simulink model "Electrical787_Isolated_2013a"  (R2013a)
settings: Solver=ode45  StartTime=0.0  StopTime=1000  RelTol=1e-3
libraries: PowerFlowLib x27, simulink x4
(part 1 of 2)
settings Model: CovModelRefEnable=off  Creator=Andrew  LastModifiedBy=Andrew
settings DataIOCC: SaveFormat=StructureWithTime
settings DebuggingCC: UnderspecifiedInitializationDetection=Simplified  MergeDetectMultiDrivingBlocksExec=error  SolverPrmCheckMsg=none  FrameProcessingCompatibilityMsg=error  StateNameClashWarn=none
settings HardwareCC: ProdBitPerPointer=64  ProdLargestAtomicFloat=Float  ProdIntDivRoundTo=Zero  ProdEndianess=LittleEndian  ProdHWDeviceType=Specified
settings GRTTargetCC: CodeReplacementLibrary=C89/C90 (ANSI)  GeneratePreprocessorConditionals=Use local settings

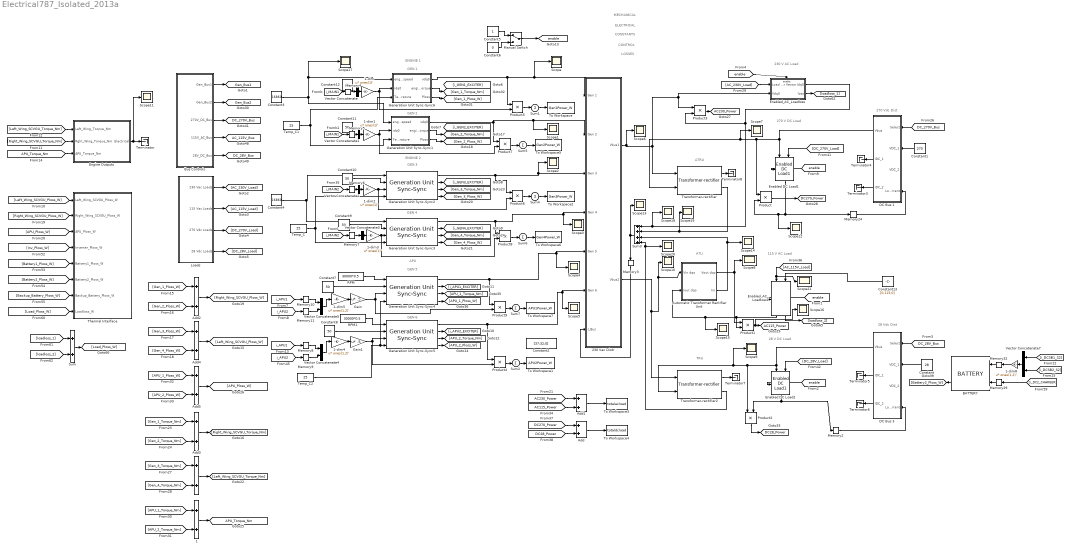
== system Electrical787_Isolated_2013a ==
  note: GEN 1
  note: ENGINE 1
  note: GEN 2
  note: GEN 3
  note: ENGINE 2
  note: GEN 4
  note: GEN 5
  note: APU
  note: GEN 6
  note: ATRU
  note: TRU
  note: 230 V AC Load
  note: 270 Vdc Dist
  note: 28 Vdc Dist
  note: 270 V DC Load
  note: CONSTANTS
  note: CONTROL
  note: LOSSES
  note: MECHANICAL
  note: ELECTRICAL
  note: ATU
  note: 115 V AC Load
  note: 28 V DC Load
  " " : Sum
  " 1" : Sum
  1-dim{,1..3} (4 alike) : Gain  Gain=ones(1)'  Multiplication=Matrix(u*K)
  1-dim4 : Gain  Gain=ones(1,2)'  Multiplication=Matrix(u*K)
  1-dim5 : Gain  Gain=ones(1,2)'  Multiplication=Matrix(u*K)
  1-dim8 : Gain  Gain=ones(1,2)'  Multiplication=Matrix(u*K)
  230 Vac Distr : Subsystem
  Add{,1..5} (6 alike) : Sum
  Automatic Transformer Rectifier Unit : Subsystem
  BATTERY : PowerFlowLib/Energy & Power Systems/Electrical/Battery/BATTERY  NO_CELLS=9  NO_MODULES=10  INITIAL_SOC=1
  Bus Controls : Subsystem  mask{BUS1=Generator 1, BUS2=Generator 2, MBUS1=Generator Bus 1, ACTBUS1=Generator Bus 1, MBUS2=Generator Bus 2, ACTBUS2=Generator Bus 2, IDCBUS1=Battery 1, IDCBUS2=Battery 2}
      mask prompts: BUS1 "Source for Bus 1"; BUS2 "Source for Bus 2"; MBUS1 "Load on Main Bus 1 drawn from"; ACTBUS1 "Load on AC Transfer Bus 1 drawn from"; MBUS2 "Load on Main Bus 2 drawn from"; ACTBUS2 "Load on AC Transfer Bus 2 drawn from"; IDCBUS1 "Source for DC Service Bus 1"; IDCBUS2 "Source for DC Service Bus 2"
      mask help:
      | Specify the source from which different buses receive power. There are
      | 1. Two Generator buses (Bus 1-2)
      | 2. Two AC Main buses (Main Bus 1-2))
      | 3. Two AC Transfer buses and (AC Transfer Bus 1-2)
      | 4. Two DC Intermediate buses (DC Intermediate Bus 1-2)
      mask init:
      | switch BUS1
      |     case 1
      |         BUS1CONTROL = 1;
      |     case 2
      |         BUS1CONTROL = 2;
      |     case 3
      |         BUS1CONTROL = 3;
      |     case 4
      |         BUS1CONTROL = 4;
      | end
      | 
      | switch BUS2
      |     case 1
      |         BUS2CONTROL = 1;
      |     case 2
      |         BUS2CONTROL = 2;
      |     case 3
      |         BUS2CONTROL = 3;
      |     case 4
      |         BUS2CONTROL = 4;
      | end
      | 
      | switch MBUS1
      |     case 1
      |         MBUS1CONTROL = 1;
      |     case 2
      |         MBUS1CONTROL = 2;
      | end
      | 
      | switch ACTBUS1
      |     case 1
      |         ACTBUS1CONTROL = 1;
      |     case 2
      |         ACTBUS1CONTROL = 2;
      | end
      | 
      | switch MBUS2
      |     case 1
      |         MBUS2CONTROL = 1;
      |     case 2
      |         MBUS2CONTROL = 2;
      | end
      | 
      | switch ACTBUS2
      |     case 1
      |         ACTBUS2CONTROL = 1;
      |     case 2
      |         ACTBUS2CONTROL = 2;
      | end
      | 
      | switch IDCBUS1
      |     case 1
      |         IDCBUS1CONTROL = 1;
      |     case 2
      |         IDCBUS1CONTROL = 2;
      | end
      | 
      | switch IDCBUS2
      |     case 1
      |         IDCBUS2CONTROL = 1;
      |     case 2
      |         IDCBUS2CONTROL = 2;
      | end
      mask TypeOptions BUS1: Generator 1  | APU  | GND | AUX SUPPLY
      mask TypeOptions BUS2: Generator 2  | APU  | GND | AUX SUPPLY
      mask TypeOptions MBUS1: Generator Bus 1 | Generator Bus 2
      mask TypeOptions ACTBUS1: Generator Bus 1 | Generator Bus 2
      mask TypeOptions MBUS2: Generator Bus 1 | Generator Bus 2
      mask TypeOptions ACTBUS2: Generator Bus 1 | Generator Bus 2
      mask TypeOptions IDCBUS1: Battery 1 | Battery 2
      mask TypeOptions IDCBUS2: Battery 1 | Battery 2
  Constant : Constant  Value=28
  Constant1 : Constant  Value=270
  Constant{7..12} (6 alike) : Constant  Value=50
  Constant13 : Constant  Value=[0,115,0]
  Constant2 : Constant  Value=[37;32;0]
  Constant3 : Constant  Value=16860
  Constant4 : Constant  Value=16860
  Constant5 : Constant
  Constant6 : Constant  Value=0
  DC Bus 1 : Subsystem  mask(DC Service Bus){}
      mask help: Service Bus
  DC Bus 3 : Subsystem  mask(DC Service Bus){}
      mask help: Service Bus
  Enabled DC Load1 : PowerFlowLib/Energy & Power Systems/Electrical/Loads/Enabled  DC Load1
  Enabled DC Load2 : PowerFlowLib/Energy & Power Systems/Electrical/Loads/Enabled  DC Load1
  Enabled_AC_Loadloss : Subsystem  AncestorBlock=PowerFlowLib/Energy & Power Systems/Electrical/Loads/Enabled_AC_Loadloss  mask(AC Loads){P=500, PF=0.85, ILRMS=0, R=10000, X=10000}
      mask prompts: P "Real Power (W)"; PF "Power factor (Range: 0 -1) : Prefix '-' sign for Cap loads"; ILRMS "Current Loading"; R "Resistance (Ohms)"; X "Reactance (Ohms)"
      mask help:
      | Enabled AC Load System.
      | Note:
      | Load Master Vector input is 1x3 matrix representing (P[W] Q[Var] I[A])
      | Extra load can be input in the boxes below and will be added with the Load Master Vector.
      mask Help: eval('open(''AC Loads_help.html'')');
      mask Callback PF:
      | blk = gcb;
      | PF    = str2num(get_param(blk,'PF'));
      | 
      | if ((PF>1) | (PF<-1))
      |    g = warndlg('Power factor magnitude should be between 0 and 1 . Reverting to default value 1','Error1','CreateMode');
      |    set_param(blk,'PF','1');
      |    open_system(blk,'mask');
      | end
      | 
      | clear g PF blk
      mask Callback X:
      | blk = gcb;
      | value1 = str2num(get_param(blk,'R'));
      | value2 = str2num(get_param(blk,'X'));
      | % eff    = str2num(get_param(blk,'E'));
      | 
      | if (value1==0) && (value2==0)
      |   h = warndlg('Both R and X cannot be 0. Reverting to default values','Error','CreateMode');
      |   set_param(blk,'R','10000');
      |   set_param(blk,'X','10000');
      | %   if ishandle(h)
      | %       close(h)
      |   open_system(blk,'mask');
      | end
      | 
      | % if ((eff>1) | (eff<0))
      | %    g = warndlg('Efficiency should be between 0 and 1 . Reverting to default value 1','Error1','CreateMode');
      | %    set_param(blk,'E','1');
      | %    open_system(blk,'mask');
      | % end
      | 
      | clear h eff blk value1 value2
      mask Display:
      | %image(imread('ACload.png'))
      | 
      | % port_label('input',1,'{\bf EXT LOAD VECTOR}','TexMode','on')
      | % port_label('input',2,'{\bf Vdq0}','TexMode','on')
      | %
      | % port_label('output',1,'{\bf Idq0}','TexMode','on')
      | % port_label('output',2,'{\bf PLOSS}','TexMode','on')
      | 
      | image(imread('ACloads.png'))
      | 
      | port_label('input',1,'{\bf Load}','TexMode','on')
      | port_label('input',2,'{\bf V_d_q_0}','TexMode','on')
      | port_label('Enable','{\bf switch}','Texmode','on')
      | 
      | port_label('output',1,'{\bf I_d_q_0}','TexMode','on')
      | port_label('output',2,'{\bf P_l_o_s_s}','TexMode','on')
  Enabled_AC_Loadloss1 : PowerFlowLib/Energy & Power Systems/Electrical/Loads/Enabled_AC_Loadloss  P=500  PF=0.85  ILRMS=0  R=10000  X=10000
  Engine Outputs : Subsystem
  Gain : Gain  Gain=.5  Multiplication=Matrix(u*K)
  Gain1 : Gain  Gain=.5  Multiplication=Matrix(u*K)
  Generation Unit Sync-Sync1 : Subsystem  AncestorBlock=PowerFlowLib/Energy & Power Systems/Electrical/Systems/Generation Unit Sync-Sync  mask{machine_mode=100kVA_Gen, Rs=0.0163, Xls=0.00054, Xmd=0.66176, Xmq=0.00099, R_fd=0.016, Xlfd=0.2092, R_1d=0.2047, Xl1d=0.6524, R_1q=0.0429, R_2q=0.0429, Xl1q=0.0639, Xl2q=0.0639, ws=377, RTL=0.001, XTL=0.1, KA=20, KF=0.063, T_f=0.35, TA=0.2, KE=1, TE=0.314, SB=100000, VBDQ=100, wB=377, P=6, H=0.1777, R_conv_gen=0.05, mc_gen=10000, Vnom=115, fan_load='init_fan_characteristics.mat', exciter_param='exciter.mat'}
      mask prompts: machine_mode "Machine Preset"; Rs "Stator Resistance [ohm]"; Xls "Stator Leakage Reactance [ohm]"; Xmd "Magnetizing Direct Axis Reactance [ohm]"; Xmq "Magnetizing Quadrature Axis Reactance [ohm]"; R_fd "Field Resistance [ohm]"; Xlfd "Field Leakage Reactance [ohm]"; R_1d "Transient Direct Axis Resistance [ohm]"; Xl1d "Transient Leakage Direct Axis Reactance [ohm]"; R_1q "Transient Quadrature Axis Resistance [ohm]"; R_2q "Subtransient Quadrature Axis Resistance [ohm]"; Xl1q "Transient Leakage Quadrature Axis Reactance [ohm]"; Xl2q "Subtransient Leakage Quadrature Axis Reactance [ohm]"; ws "Rotational Speed [rad/s]"; RTL "Resistance [ohm]"; XTL "Reactance [ohm]"; SB "Baes Complex Power [VA]"; VBDQ "Base Direct and Quadrature Axis Armature Voltage [V]"; wB "Base Electrical Frequency [rad/s]"; P "Number of Pole Pairs"; H "Shaft Inertia Constant [s]"; Vnom "Nominal Voltage [V]"; fan_load "Fan Load"; exciter_param "Exciter Machine Parameters"
      mask help:
      | A generator system block implements a generic power generation unit consisting of a gearbox, a synchronous generator, a synchronous exciter and exciter controls.
      | The generator size can be selected from the drop window below.
      | (For advanced-users) When the User-defined option is selected from the drop window, the generator parameters can be manually specified in the tabs below.
      |
      | Block Inputs:
      |
      | #1: Jet engine low pressure spool [RPM]
      | #2: Exciter system supply voltage [V]
      | #3: Synchronous reference frame line currents  [A]
      |
      | Block Output:
      |
      | #1: Synchronous reference frame line voltages [V]
      | #2: Exciter system supply current [A]
      | #3: Electromagnetic torque on the low pressure spool  [N-M]
      | #4: Heat rejected to the cooling system or ambient [W]
      mask init:
      | load(fan_load);
      | 
      | % Inductances
      | Xd = Xls + Xmd;
      | Xq = Xls + Xmq;
      | Xfd = Xlfd + Xmd;
      | X1q = Xl1q + Xmq;
      | Xd1 = Xd - Xmd^2/Xfd;
      | Xq1 = Xq - Xmq^2/X1q;
      | Xd2 = Xls + (1/(1/Xmd + 1/Xlfd + 1/Xl1d));
      | Xq2 = Xls + (1/(1/Xmq + 1/Xl1q + 1/Xl2q));
      | Tdo1 = Xfd/ws/R_fd;
      | Tqo1 = X1q/ws/R_1q;
      | Tdo2 = 1/ws/R_1d*(Xl1d + 1/(1/Xmd + 1/Xlfd));
      | Tqo2 = 1/ws/R_2q*(Xl2q+1/(1/Xmq + 1/Xl1q));
      | 
      | % Base Quantities
      | 
      | TB = (P/2)*SB/wB;
      | IBDQ = SB/VBDQ;
      | LBDQ = VBDQ/wB;
      | 
      | IBFD = IBDQ;
      | IB1D = IBDQ;
      | IB1Q = IBDQ;
      | IB2Q = IBDQ;
      | 
      | VBFD = SB/IBFD;
      | VB1D = SB/IB1D;
      | VB1Q = SB/IB1Q;
      | VB2Q = SB/IB2Q;
      | 
      | LBFD = VBFD/wB;
      | LB1D = VB1D/wB;
      | LB1Q = VB1Q/wB;
      | LB2Q = VB2Q/wB;
      | 
      | J = 2*H/(wB*2/P)^2*SB;
      | M = 2*H/wB;
      | 
      | % Exciter
      | 
      | data_exc = load(exciter_param);
      |   
      | % Stator
      | Rs_exc = data_exc.r(1);
      | Xls_exc = data_exc.r(2);
      | Xmd_exc = data_exc.r(3);
      | Xmq_exc = data_exc.r(4);
      | 
      | % Field
      | R_fd_exc = data_exc.r(5);
      | Xlfd_exc = data_exc.r(6);
      | % Dampers
      | R_1d_exc = data_exc.r(7);
      | Xl1d_exc = data_exc.r(8);
      | R_1q_exc = data_exc.r(9);
      | Xl1q_exc = data_exc.r(10);
      | R_2q_exc = data_exc.r(11);
      | Xl2q_exc = data_exc.r(12);
      | 
      | % Rotor
      | P_exc = data_exc.r(13);
      | ws_exc = data_exc.r(14);
      | 
      | % Inductances
      | Xd_exc = Xls_exc + Xmd_exc;
      | Xq_exc = Xls_exc + Xmq_exc;
      | Xfd_exc = Xlfd_exc + Xmd_exc;
      | X1q_exc = Xl1q_exc + Xmq_exc;
      | Xd1_exc = Xd_exc - Xmd_exc^2/Xfd_exc;
      | Xq1_exc = Xq_exc - Xmq_exc^2/X1q_exc;
      | Xd2_exc = Xls_exc + (1/(1/Xmd_exc + 1/Xlfd_exc + 1/Xl1d_exc));
      | Xq2_exc = Xls_exc + (1/(1/Xmq_exc + 1/Xl1q_exc + 1/Xl2q_exc));
      | Tdo1_exc = Xfd_exc/ws_exc/R_fd_exc;
      | Tqo1_exc = X1q_exc/ws_exc/R_1q_exc;
      | Tdo2_exc = 1/ws_exc/R_1d_exc*(Xl1d_exc + 1/(1/Xmd_exc + 1/Xlfd_exc));
      | Tqo2_exc = 1/ws_exc/R_2q_exc*(Xl2q_exc+1/(1/Xmq_exc + 1/Xl1q_exc));
      | 
      | % Transmission Line
      | RTL_exc = data_exc.r(15);
      | XTL_exc = data_exc.r(16);
      | 
      | % Regulator and Governor
      | KA_exc = data_exc.r(17);
      | KF_exc = data_exc.r(18);
      | T_f_exc = data_exc.r(19);
      | TA_exc = data_exc.r(20);
      | KE_exc = data_exc.r(21);
      | TE_exc = data_exc.r(22);
      | 
      | % Base Quantities
      | SB_exc = data_exc.r(23);
      | VBDQ_exc = data_exc.r(24);
      | wB_exc = data_exc.r(25);
      | P_exc = data_exc.r(13);
      | H_exc = data_exc.r(26);
      | 
      | TB_exc = (P/2)*SB_exc/wB_exc;
      | IBDQ_exc = SB_exc/VBDQ_exc;
      | LBDQ_exc = VBDQ_exc/wB_exc;
      | 
      | IBFD_exc = IBDQ_exc;
      | IB1D_exc = IBDQ_exc;
      | IB1Q_exc = IBDQ_exc;
      | IB2Q_exc = IBDQ_exc;
      | 
      | VBFD_exc = SB_exc/IBFD_exc;
      | VB1D_exc = SB_exc/IB1D_exc;
      | VB1Q_exc = SB_exc/IB1Q_exc;
      | VB2Q_exc = SB_exc/IB2Q_exc;
      | 
      | LBFD_exc = VBFD_exc/wB_exc;
      | LB1D_exc = VB1D_exc/wB_exc;
      | LB1Q_exc = VB1Q_exc/wB_exc;
      | LB2Q_exc = VB2Q_exc/wB_exc;
      | 
      | J_exc = 2*data_exc.r(26)/(wB_exc*2/P_exc)^2*SB_exc;
      | M_exc = 2*H_exc/wB_exc;
      | 
      | R_conv_gen_exc = 1/data_exc.r(27);
      | mc_gen_exc = data_exc.r(28);
      mask Help: eval('open(''Generator System_help.html'')');
      mask TypeOptions machine_mode: 20kVA_Gen | 52.5kVA_Gen | 100kVA_Gen | 300kVA_Gen | 800kVA_Gen | 1MVA_Gen | User-defined
      mask Callback machine_mode:
      | h=get_param(gcb,'handle');
      | hblock=get(h);
      | data=load('GenProp.mat');
      | 
      | if strcmp(hblock.machine_mode,'User-defined')==1;
      |     adv_warn=warndlg(sprintf('User-defined parameters may lead to an unstable build.'));
      | 
      |     % grabs current values of enabled GUI parameters
      |     mskenabl = get_param(gcb,'MaskEnables');
      |     mskenabl(1:size(mskenabl,1)) = {'on'};  % sets all parameters to enable
      |     set_param(gcb,'MaskEnables',mskenabl)
      | 
      | else
      |     % For each generator preset references a column from GenProp.mat
      |     if strcmp(hblock.machine_mode,'20kVA_Gen')==1; n=1;
      |     elseif strcmp(hblock.machine_mode,'52.5kVA_Gen')==1; n=2;
      |     elseif strcmp(hblock.machine_mode,'100kVA_Gen')==1; n=3;
      |     elseif strcmp(hblock.machine_mode,'300kVA_Gen')==1; n=4;
      |     elseif strcmp(hblock.machine_mode,'800kVA_Gen')==1; n=5;
      |     elseif strcmp(hblock.machine_mode,'1MVA_Gen')==1; n=6;
      |     end
      |     % Set each parameter of the generator
      |     set1=num2str(data.r(1,n));
      |     set2=num2str(data.r(2,n));
      |     set3=num2str(data.r(3,n));
      |     set4=num2str(data.r(4,n));
      |     set_param(gcb,'Rs',set1,'Xls',set2,'Xmd',set3,'Xmq',set4)
      |     set1=num2str(data.r(5,n));
      |     set2=num2str(data.r(6,n));
      |     set_param(gcb,'R_fd',set1,'Xlfd',set2) %5 and 6
      |     set1=num2str(data.r(7,n));
      |     set2=num2str(data.r(8,n));
      |     set3=num2str(data.r(9,n));
      |     set4=num2str(data.r(10,n));
      |     set5=num2str(data.r(11,n));
      |     set6=num2str(data.r(12,n));
      |     set_param(gcb,'R_1d',set1,'Xl1d',set2,'R_1q',set3,'Xl1q',set4,'R_2q',set5,'Xl2q',set6) %7-12
      |     set1=num2str(data.r(14,n));
      |     set2=num2str(data.r(15,n));
      |     set3=num2str(data.r(16,n));
      |     set_param(gcb,'ws',set1,'RTL',set2,'XTL',set3)
      |     set1=num2str(data.r(17,n));
      |     set2=num2str(data.r(18,n));
      |     set3=num2str(data.r(19,n));
      |     set4=num2str(data.r(20,n));
      |     set5=num2str(data.r(21,n));
      |     set6=num2str(data.r(22,n));
      |     set_param(gcb,'KA',set1,'KF',set2,'T_f',set3,'TA',set4,'KE',set5,'TE',set6)
      |     set1=num2str(data.r(23,n));
      |     set2=num2str(data.r(24,n));
      |     set3=num2str(data.r(25,n));
      |     set4=num2str(data.r(13,n));
      |     set5=num2str(data.r(26,n));
      |     set_param(gcb,'SB',set1,'VBDQ',set2,'wB',set3,'P',set4,'H',set5)
      |     set1=num2str(1/data.r(27,n));
      |     set2=num2str(data.r(28,n));
      |     set_param(gcb,'R_conv_gen',set1,'mc_gen',set2)
      | 
      |     % grabs current values of enabled GUI parameters
      |     mskenabl = get_param(gcb,'MaskEnables');
      |     % sets all parameters to enable
      |     mskenabl(2:size(mskenabl,1)-3) = {'off'};
      |     set_param(gcb,'MaskEnables',mskenabl)
      | 
      | 
      | end
      | 
      | 
      | clear h hblock n data mskenabl
      | clear set1 set2 set3 set4 set5 set6
      mask Display:
      | image(imread('Generator.png')) % Load image
      | 
      | % Define inputs
      | 
      | port_label('input',1,'{\bf \omega_s_h_a_f_t}','Texmode','on')
      | port_label('input',2,'{\bf V_D_C}','Texmode','on')
      | port_label('input',3,'{\bf I_d_q_0}','Texmode','on')
      | port_label('input',4,'{\bf Temp}','Texmode','on')
      | 
      | % Define outputs
      | 
      | port_label('output',1,'{\bf V_d_q_0}','Texmode','on')
      | port_label('output',2,'{\bf I_D_C}','Texmode','on')
      | port_label('output',3,'{\bf \tau}','Texmode','on')
      | port_label('output',4,'{\bf P_l_o_s_s}','Texmode','on')
      | 
      | % % Define inputs
      | %
      | % port_label('input',1,'{\bf Generator Speed}','Texmode','on')
      | % port_label('input',2,'{\bf Battery Voltage}','Texmode','on')
      | % port_label('input',3,'{\bf Line Currents}','Texmode','on')
      | %
      | % % Define outputs
      | %
      | % port_label('output',1,'{\bf Line Voltages}','Texmode','on')
      | % port_label('output',2,'{\bf Battery Current}','Texmode','on')
      | % port_label('output',3,'{\bf Generator Torque}','Texmode','on')
      | % port_label('output',4,'{\bf Power Loss}','Texmode','on')
  Generation Unit Sync-Sync{2..5} (4 alike) : PowerFlowLib/Energy & Power Systems/Electrical/Systems/Generation Unit Sync-Sync  machine_mode=100kVA_Gen  Rs=0.0163  Xls=0.00054  Xmd=0.66176  Xmq=0.00099  R_fd=0.016  Xlfd=0.2092  R_1d=0.2047  Xl1d=0.6524  R_1q=0.0429  R_2q=0.0429  Xl1q=0.0639  Xl2q=0.0639  ws=377  RTL=0.001  XTL=0.1  KA=20  KF=0.063  T_f=0.35  TA=0.2  KE=1  TE=0.314  SB=100000  VBDQ=100  wB=377  P=6  H=0.1777  R_conv_gen=0.05  mc_gen=10000  Vnom=115  fan_load='init_fan_characteristics.mat'  exciter_param='exciter.mat'
  Generation Unit Sync-Sync6 : Subsystem  AncestorBlock=PowerFlowLib/Energy & Power Systems/Electrical/Systems/Generation Unit Sync-Sync  mask{machine_mode=100kVA_Gen, Rs=0.0163, Xls=0.00054, Xmd=0.66176, Xmq=0.00099, R_fd=0.016, Xlfd=0.2092, R_1d=0.2047, Xl1d=0.6524, R_1q=0.0429, R_2q=0.0429, Xl1q=0.0639, Xl2q=0.0639, ws=377, RTL=0.001, XTL=0.1, KA=20, KF=0.063, T_f=0.35, TA=0.2, KE=1, TE=0.314, SB=100000, VBDQ=100, wB=377, P=6, H=0.1777, R_conv_gen=0.05, mc_gen=10000, Vnom=115, fan_load='init_fan_characteristics.mat', exciter_param='exciter.mat'}
      mask prompts: machine_mode "Machine Preset"; Rs "Stator Resistance [ohm]"; Xls "Stator Leakage Reactance [ohm]"; Xmd "Magnetizing Direct Axis Reactance [ohm]"; Xmq "Magnetizing Quadrature Axis Reactance [ohm]"; R_fd "Field Resistance [ohm]"; Xlfd "Field Leakage Reactance [ohm]"; R_1d "Transient Direct Axis Resistance [ohm]"; Xl1d "Transient Leakage Direct Axis Reactance [ohm]"; R_1q "Transient Quadrature Axis Resistance [ohm]"; R_2q "Subtransient Quadrature Axis Resistance [ohm]"; Xl1q "Transient Leakage Quadrature Axis Reactance [ohm]"; Xl2q "Subtransient Leakage Quadrature Axis Reactance [ohm]"; ws "Rotational Speed [rad/s]"; RTL "Resistance [ohm]"; XTL "Reactance [ohm]"; SB "Baes Complex Power [VA]"; VBDQ "Base Direct and Quadrature Axis Armature Voltage [V]"; wB "Base Electrical Frequency [rad/s]"; P "Number of Pole Pairs"; H "Shaft Inertia Constant [s]"; Vnom "Nominal Voltage [V]"; fan_load "Fan Load"; exciter_param "Exciter Machine Parameters"
      mask help:
      | A generator system block implements a generic power generation unit consisting of a gearbox, a synchronous generator, a synchronous exciter and exciter controls.
      | The generator size can be selected from the drop window below.
      | (For advanced-users) When the User-defined option is selected from the drop window, the generator parameters can be manually specified in the tabs below.
      |
      | Block Inputs:
      |
      | #1: Jet engine low pressure spool [RPM]
      | #2: Exciter system supply voltage [V]
      | #3: Synchronous reference frame line currents  [A]
      |
      | Block Output:
      |
      | #1: Synchronous reference frame line voltages [V]
      | #2: Exciter system supply current [A]
      | #3: Electromagnetic torque on the low pressure spool  [N-M]
      | #4: Heat rejected to the cooling system or ambient [W]
      mask init: same as Electrical787_Isolated_2013a/Generation Unit Sync-Sync1
      mask Help: eval('open(''Generator System_help.html'')');
      mask TypeOptions machine_mode: 20kVA_Gen | 52.5kVA_Gen | 100kVA_Gen | 300kVA_Gen | 800kVA_Gen | 1MVA_Gen | User-defined
      mask Callback machine_mode:
      | h=get_param(gcb,'handle');
      | hblock=get(h);
      | data=load('GenProp.mat');
      | 
      | if strcmp(hblock.machine_mode,'User-defined')==1;
      |     adv_warn=warndlg(sprintf('User-defined parameters may lead to an unstable build.'));
      | 
      |     % grabs current values of enabled GUI parameters
      |     mskenabl = get_param(gcb,'MaskEnables');
      |     mskenabl(1:size(mskenabl,1)) = {'on'};  % sets all parameters to enable
      |     set_param(gcb,'MaskEnables',mskenabl)
      | 
      | else
      |     % For each generator preset references a column from GenProp.mat
      |     if strcmp(hblock.machine_mode,'20kVA_Gen')==1; n=1;
      |     elseif strcmp(hblock.machine_mode,'52.5kVA_Gen')==1; n=2;
      |     elseif strcmp(hblock.machine_mode,'100kVA_Gen')==1; n=3;
      |     elseif strcmp(hblock.machine_mode,'300kVA_Gen')==1; n=4;
      |     elseif strcmp(hblock.machine_mode,'800kVA_Gen')==1; n=5;
      |     elseif strcmp(hblock.machine_mode,'1MVA_Gen')==1; n=6;
      |     end
      |     % Set each parameter of the generator
      |     set1=num2str(data.r(1,n));
      |     set2=num2str(data.r(2,n));
      |     set3=num2str(data.r(3,n));
      |     set4=num2str(data.r(4,n));
      |     set_param(gcb,'Rs',set1,'Xls',set2,'Xmd',set3,'Xmq',set4)
      |     set1=num2str(data.r(5,n));
      |     set2=num2str(data.r(6,n));
      |     set_param(gcb,'R_fd',set1,'Xlfd',set2) %5 and 6
      |     set1=num2str(data.r(7,n));
      |     set2=num2str(data.r(8,n));
      |     set3=num2str(data.r(9,n));
      |     set4=num2str(data.r(10,n));
      |     set5=num2str(data.r(11,n));
      |     set6=num2str(data.r(12,n));
      |     set_param(gcb,'R_1d',set1,'Xl1d',set2,'R_1q',set3,'Xl1q',set4,'R_2q',set5,'Xl2q',set6) %7-12
      |     set1=num2str(data.r(14,n));
      |     set2=num2str(data.r(15,n));
      |     set3=num2str(data.r(16,n));
      |     set_param(gcb,'ws',set1,'RTL',set2,'XTL',set3)
      |     set1=num2str(data.r(17,n));
      |     set2=num2str(data.r(18,n));
      |     set3=num2str(data.r(19,n));
      |     set4=num2str(data.r(20,n));
      |     set5=num2str(data.r(21,n));
      |     set6=num2str(data.r(22,n));
      |     set_param(gcb,'KA',set1,'KF',set2,'T_f',set3,'TA',set4,'KE',set5,'TE',set6)
      |     set1=num2str(data.r(23,n));
      |     set2=num2str(data.r(24,n));
      |     set3=num2str(data.r(25,n));
      |     set4=num2str(data.r(13,n));
      |     set5=num2str(data.r(26,n));
      |     set_param(gcb,'SB',set1,'VBDQ',set2,'wB',set3,'P',set4,'H',set5)
      |     set1=num2str(1/data.r(27,n));
      |     set2=num2str(data.r(28,n));
      |     set_param(gcb,'R_conv_gen',set1,'mc_gen',set2)
      | 
      |     % grabs current values of enabled GUI parameters
      |     mskenabl = get_param(gcb,'MaskEnables');
      |     % sets all parameters to enable
      |     mskenabl(2:size(mskenabl,1)-3) = {'off'};
      |     set_param(gcb,'MaskEnables',mskenabl)
      | 
      | 
      | end
      | 
      | 
      | clear h hblock n data mskenabl
      | clear set1 set2 set3 set4 set5 set6
      mask Display:
      | image(imread('Generator.png')) % Load image
      | 
      | % Define inputs
      | 
      | port_label('input',1,'{\bf \omega_s_h_a_f_t}','Texmode','on')
      | port_label('input',2,'{\bf V_D_C}','Texmode','on')
      | port_label('input',3,'{\bf I_d_q_0}','Texmode','on')
      | port_label('input',4,'{\bf Temp}','Texmode','on')
      | 
      | % Define outputs
      | 
      | port_label('output',1,'{\bf V_d_q_0}','Texmode','on')
      | port_label('output',2,'{\bf I_D_C}','Texmode','on')
      | port_label('output',3,'{\bf \tau}','Texmode','on')
      | port_label('output',4,'{\bf P_l_o_s_s}','Texmode','on')
      | 
      | % % Define inputs
      | %
      | % port_label('input',1,'{\bf Generator Speed}','Texmode','on')
      | % port_label('input',2,'{\bf Battery Voltage}','Texmode','on')
      | % port_label('input',3,'{\bf Line Currents}','Texmode','on')
      | %
      | % % Define outputs
      | %
      | % port_label('output',1,'{\bf Line Voltages}','Texmode','on')
      | % port_label('output',2,'{\bf Battery Current}','Texmode','on')
      | % port_label('output',3,'{\bf Generator Torque}','Texmode','on')
      | % port_label('output',4,'{\bf Power Loss}','Texmode','on')
  Loads : Subsystem
  Manual Switch : ManualSwitch
  Memory{2..11,24,29,32} (13 alike) : Memory
  Product{,1..9} (10 alike) : Product
  RPM : Constant  Value=30000*0.5
  RPM1 : Constant  Value=30000*0.5
  Scope{,1..21} (22 alike) : Scope
      Scope settings: ShowLegends=on  YMin=-1.15008  YMax=10.35076
      Scope1 settings: ShowLegends=on  YMin=-1.15008  YMax=10.35076
      Scope10 settings: ShowLegends=on  YMin=-14.375  YMax=129.375  SaveName=ScopeData10
      Scope11 settings: ShowLegends=on  YMin=-10  YMax=10  SaveName=ScopeData11
      Scope12 settings: ShowLegends=on  YMin=50.00000  YMax=250.00000  SaveName=ScopeData12
      Scope13 settings: ShowLegends=on  YMin=0.38349  YMax=34.27475  SaveName=ScopeData13
      Scope14 settings: ShowLegends=on  YMin=-1.00000  YMax=1.00000  SaveName=ScopeData24
      Scope15 settings: ShowLegends=on  YMin=-0.33753  YMax=3.0378  SaveName=ScopeData26
      Scope16 settings: ShowLegends=on  YMin=-0.000000000000003  YMax=0.000000000000029  SaveName=ScopeData30
      Scope17 settings: ShowLegends=on  YMin=-2.15456  YMax=19.34868  SaveName=ScopeData31
      Scope18 settings: YMin=-4.205  YMax=37.84499  SaveName=ScopeData3
      Scope19 settings: YMin=-1.00000  YMax=1.00000  SaveName=ScopeData4
      Scope2 settings: ShowLegends=on  YMin=-0.000000000000000000011  YMax=0.000000000000000000077  SaveName=ScopeData2
      Scope20 settings: YMin=-1.00000  YMax=1.00000  SaveName=ScopeData5
      Scope21 settings: ShowLegends=on  YMin=-18.75  YMax=168.75  SaveName=ScopeData6
      Scope3 settings: ShowLegends=on  YMin=-14.375  YMax=129.375  SaveName=ScopeData3
      Scope4 settings: ShowLegends=on  YMin=-14.375  YMax=129.375  SaveName=ScopeData4
      Scope5 settings: ShowLegends=on  YMin=-1.00000  YMax=1.00000  SaveName=ScopeData5
      Scope6 settings: ShowLegends=on  YMin=-14.46445  YMax=130.17984  SaveName=ScopeData6
      Scope7 settings: ShowLegends=on  YMin=170.00000  YMax=370.00000  SaveName=ScopeData7
      Scope8 settings: ShowLegends=on  YMin=-4.7826  YMax=43.04342  SaveName=ScopeData8
      Scope9 settings: ShowLegends=on  YMin=18.00000  YMax=38.00000  SaveName=ScopeData9
  Sum : Sum
  Sum{1..2,4..7} (6 alike) : Sum  Inputs=+
  Sum3 : Sum  Inputs=++++
  Temp_C : Constant  Value=25
  Temp_C1 : Constant  Value=25
  Temp_C2 : Constant  Value=25
  Terminator{,3..8} (7 alike) : Terminator
  Thermal Interface : Subsystem
  To Workspace : ToWorkspace  VariableName=Gen1Power_W  SampleTime=10  SaveFormat=Structure With Time
  To Workspace1 : ToWorkspace  VariableName=APU2Power_W  SampleTime=10  SaveFormat=Structure With Time
  To Workspace2 : ToWorkspace  VariableName=Gen3Power_W  SampleTime=10  SaveFormat=Structure With Time
  To Workspace3 : ToWorkspace  VariableName=totalacload  SampleTime=-1  SaveFormat=Timeseries
  To Workspace4 : ToWorkspace  VariableName=totaldcload  SampleTime=-1  SaveFormat=Timeseries
  To Workspace5 : ToWorkspace  VariableName=Gen2Power_W  SampleTime=10  SaveFormat=Structure With Time
  To Workspace6 : ToWorkspace  VariableName=Gen4Power_W  SampleTime=10  SaveFormat=Structure With Time
  To Workspace7 : ToWorkspace  VariableName=APU1Power_W  SampleTime=10  SaveFormat=Structure With Time
  Transformer-rectifier : PowerFlowLib/Energy & Power Systems/Electrical/Systems/Transformer-rectifier  pu=1
      link override Transformer1: N2=332
  Transformer-rectifier2 : PowerFlowLib/Energy & Power Systems/Electrical/Systems/Transformer-rectifier  pu=1
      link override Transformer1: N2=34
  Vector Concatenate{,1..3} (4 alike) : Concatenate  NumInputs=1  Mode=Multidimensional array  ConcatenateDimension=2
  Vector Concatenate4 : Concatenate  Mode=Multidimensional array  ConcatenateDimension=2
  Vector Concatenate5 : Concatenate  Mode=Multidimensional array  ConcatenateDimension=2
  Vector Concatenate7 : Concatenate  Mode=Multidimensional array  ConcatenateDimension=2
  tag scope: AC115_Power=global, AC230_Power=global, AC_115V_Bus=global, APU_Torque_Nm=global, DC270_Power=global, DC28_Power=global, DC_270V_Bus=global, DC_28V_Bus=global, Gen_Bus1=global, Gen_Bus2=global, enable=global
  wires:
  Generation Unit Sync-Sync6/1(vdq0) -> Product5/1, Scope/1, 230 Vac Distr/1(Gen 1)
  Generation Unit Sync-Sync1/1(vdq0) -> Scope1/1, 230 Vac Distr/2(Gen 2), Product7/1
  Generation Unit Sync-Sync2/1 -> Product6/1, Scope2/1, 230 Vac Distr/3(Gen 3)
  Generation Unit Sync-Sync3/1 -> Product8/1, Scope3/1, 230 Vac Distr/4(Gen 4)
  Generation Unit Sync-Sync4/1 -> Product9/1, Scope4/1, 230 Vac Distr/5(Gen 5)
  Generation Unit Sync-Sync5/1 -> Product4/1, Scope5/1, 230 Vac Distr/6(Gen 6)
  230 Vac Distr/1(Vbus1) -> Enabled_AC_Loadloss/2(Vdq0), Product3/1, Transformer-rectifier/1, Scope6/1
  230 Vac Distr/2(Vbus2) -> Transformer-rectifier2/1, Scope10/1, Automatic Transformer Rectifier Unit/1(Vin dqo)
  [enable] -> Enabled_AC_Loadloss/Enable
  DC Bus 1/1(Vbus) -> Scope7/1, Transformer-rectifier/2, Product/1, Enabled DC Load1/1
  DC Bus 3/1(Vbus) -> Enabled DC Load2/1, Product2/1, Scope9/1, Transformer-rectifier2/2
  Enabled DC Load1/1 -> Scope12/1, Product/2, Memory24/1
  Memory24/1 -> DC Bus 1/4(Load current)
  Enabled DC Load2/1 -> Product2/2, Memory2/1
  Memory2/1 -> DC Bus 3/4(Load current)
  [enable] -> Enabled DC Load1/Enable
  [enable] -> Enabled_AC_Loadloss1/Enable
  [enable] -> Enabled DC Load2/Enable
  Transformer-rectifier2/2 -> Scope20/1, Sum3/4
  Transformer-rectifier/2 -> Scope19/1, Sum3/2
  Enabled_AC_Loadloss/1(Idq0) -> Product3/2, Scope18/1, Sum3/1
  Sum3/1 -> Scope13/1, Memory3/1
  Enabled_AC_Loadloss1/1 -> Scope15/1, Automatic Transformer Rectifier Unit/2(Iout dqo), Product1/2
  Memory32/1 -> BATTERY/1
  1-dim8/1 -> Memory32/1
  [i_DCSB1_S2] -> Vector Concatenate7/1
  [i_DCSB2_S2] -> Vector Concatenate7/2
  Vector Concatenate7/1 -> 1-dim8/1
  Memory29/1 -> BATTERY/2
  [i_DC2_CHARGER] -> Memory29/1
  [AC_230V_Load] -> Enabled_AC_Loadloss/1(Load Master Vector)
  Enabled_AC_Loadloss/2(loss) -> [loadloss_1]
  Add/1 -> To Workspace4/1
  Add1/1 -> To Workspace3/1
  Enabled_AC_Loadloss1/2 -> [loadloss_2]
  [AC_115V_Load] -> Scope21/1, Enabled_AC_Loadloss1/1
  [DC_270V_Load] -> Enabled DC Load1/2
  Loads/1(230 Vac Loads) -> [AC_230V_Load]
  Loads/2(115 Vac Loads) -> [AC_115V_Load]
  Loads/3(270 Vdc Loads) -> [DC_270V_Load]
  Loads/4(28 Vdc Loads) -> [DC_28V_Load]
  [DC_270V_Bus] -> DC Bus 1/1(Select)
  [DC_28V_Bus] -> DC Bus 3/1(Select)
  Bus Controls/1(Gen_Bus1) -> [Gen_Bus1]
  Bus Controls/2(Gen_Bus2) -> [Gen_Bus2]
  Bus Controls/5(28V_DC_Bus) -> [DC_28V_Bus]
  BATTERY/2 -> [Battery2_Ploss_W]
  Bus Controls/4(115V_AC_Bus) -> [AC_115V_Bus]
  Bus Controls/3(270V_DC_Bus) -> [DC_270V_Bus]
  [i_MAIN1] -> Memory4/1
  [i_MAIN2] -> Memory6/1
  [i_MAIN2] -> Memory7/1
  [i_MAIN1] -> Memory5/1
  Memory7/1 -> Vector Concatenate3/1
  Vector Concatenate3/1 -> 1-dim3/1
  1-dim3/1 -> Product8/2, Generation Unit Sync-Sync3/3
  Memory6/1 -> Vector Concatenate2/1
  Vector Concatenate2/1 -> 1-dim2/1
  1-dim2/1 -> Product6/2, Generation Unit Sync-Sync2/3
  Memory5/1 -> Vector Concatenate1/1
  Vector Concatenate1/1 -> 1-dim1/1
  1-dim1/1 -> Generation Unit Sync-Sync1/2(idq0), Product7/2
  Memory4/1 -> Vector Concatenate/1
  Vector Concatenate/1 -> 1-dim/1
  1-dim/1 -> Generation Unit Sync-Sync6/2(idq0), Product5/2
  Manual Switch/1 -> [enable]
  Constant3/1 -> Generation Unit Sync-Sync1/1(engine speed), Generation Unit Sync-Sync6/1(engine speed), Scope17/1
  Constant4/1 -> Generation Unit Sync-Sync3/1, Generation Unit Sync-Sync2/1
  Generation Unit Sync-Sync2/2 -> [i_GEN3_EXCITER]
  Generation Unit Sync-Sync3/2 -> [i_GEN4_EXCITER]
  Constant10/1 -> Generation Unit Sync-Sync2/2
  Constant9/1 -> Generation Unit Sync-Sync3/2
  Temp_C1/1 -> Generation Unit Sync-Sync1/3(Temperature), Generation Unit Sync-Sync6/3(Temperature)
  Temp_C/1 -> Generation Unit Sync-Sync3/4, Generation Unit Sync-Sync2/4
  Product4/1 -> Sum2/1
  Sum2/1 -> To Workspace1/1
  Vector Concatenate4/1 -> 1-dim4/1
  [i_APU2] -> Memory9/1
  [i_APU1] -> Memory8/1
  Memory8/1 -> Vector Concatenate4/1
  Memory9/1 -> Vector Concatenate4/2
  Constant8/1 -> Generation Unit Sync-Sync5/2
  Temp_C2/1 -> Generation Unit Sync-Sync4/4, Generation Unit Sync-Sync5/4
  Vector Concatenate5/1 -> 1-dim5/1
  [i_APU2] -> Memory11/1
  [i_APU1] -> Memory10/1
  Memory10/1 -> Vector Concatenate5/1
  Memory11/1 -> Vector Concatenate5/2
  Constant7/1 -> Generation Unit Sync-Sync4/2
  Product5/1 -> Sum1/1
  Sum1/1 -> To Workspace/1
  Product6/1 -> Sum4/1
  Sum4/1 -> To Workspace2/1
  Product7/1 -> Sum5/1
  Sum5/1 -> To Workspace5/1
  Product8/1 -> Sum6/1
  Sum6/1 -> To Workspace6/1
  Product9/1 -> Sum7/1
  Sum7/1 -> To Workspace7/1
  [Left_Wing_SCVGU_Torque_Nm] -> Engine Outputs/1(Left_Wing_Toqrue_Nm)
  [Right_Wing_SCVGU_Torque_Nm] -> Engine Outputs/2(Rght_Wing_Torque_Nm)
  [APU_Torque_Nm] -> Engine Outputs/3(APU_Torque_Nm)
  [Left_Wing_SCVGU_Ploss_W] -> Thermal Interface/1(Left_Wing_SCVGU_Ploss_W)
  [Right_Wing_SCVGU_Ploss_W] -> Thermal Interface/2(Right_Wing_SCVGU_Ploss_W)
  [APU_Ploss_W] -> Thermal Interface/3(APU_Ploss_W)
  [Inv_Ploss_W] -> Thermal Interface/4(Inverter_Ploss_W)
  [Battery1_Ploss_W] -> Thermal Interface/5(Battery1_Ploss_W)
  [Battery2_Ploss_W] -> Thermal Interface/6(Battery2_Ploss_W)
  [Backup_Battery_Ploss_W] -> Thermal Interface/7(Backup_Battery_Ploss_W)
  [Load_Ploss_W] -> Thermal Interface/8(Loadloss_W)
  [loadloss_1] -> Sum/1
  [loadloss_2] -> Sum/2
  Sum/1 -> [Load_Ploss_W]
  Generation Unit Sync-Sync4/3 -> [APU_1_Torque_Nm]
  Generation Unit Sync-Sync5/3 -> [APU_2_Torque_Nm]
  Generation Unit Sync-Sync4/2 -> [i_APU1_EXCITER]
  Generation Unit Sync-Sync4/4 -> [APU_1_Ploss_W]
  Generation Unit Sync-Sync5/4 -> [APU_2_Ploss_W]
  Generation Unit Sync-Sync5/2 -> [i_APU2_EXCITER]
  Generation Unit Sync-Sync6/3(Ploss) -> [Gen_1_Ploss_W]
  Generation Unit Sync-Sync6/2(engine torque) -> [Gen_1_Torque_Nm]
  Generation Unit Sync-Sync1/2(engine torque) -> [Gen_2_Torque_Nm]
  Generation Unit Sync-Sync1/3(Ploss) -> [Gen_2_Ploss_W]
  Add4/1 -> [Left_Wing_SCVGU_Ploss_W]
  Add2/1 -> [Right_Wing_SCVGU_Ploss_W]
  [Gen_1_Ploss_W] -> Add2/1
  [Gen_2_Ploss_W] -> Add2/2
  Generation Unit Sync-Sync3/4 -> [Gen_4_Ploss_W]
  Generation Unit Sync-Sync2/4 -> [Gen_3_Ploss_W]
  [Gen_4_Ploss_W] -> Add4/2
  [Gen_3_Ploss_W] -> Add4/1
  Add3/1 -> [Right_Wing_SCVGU_Torque_Nm]
  " "/1 -> [Left_Wing_SCVGU_Torque_Nm]
  Generation Unit Sync-Sync3/3 -> [Gen_4_Torque_Nm]
  Generation Unit Sync-Sync2/3 -> [Gen_3_Torque_Nm]
  [Gen_1_Torque_Nm] -> Add3/1
  [Gen_2_Torque_Nm] -> Add3/2
  [Gen_3_Torque_Nm] -> " "/1
  [Gen_4_Torque_Nm] -> " "/2
  1-dim5/1 -> Gain/1
  Gain/1 -> Product9/2, Generation Unit Sync-Sync4/3
  Gain1/1 -> Product4/2, Generation Unit Sync-Sync5/3
  1-dim4/1 -> Gain1/1
  " 1"/1 -> [APU_Torque_Nm]
  [APU_1_Torque_Nm] -> " 1"/1
  [APU_2_Torque_Nm] -> " 1"/2
  Add5/1 -> [APU_Ploss_W]
  [APU_2_Ploss_W] -> Add5/2
  [APU_1_Ploss_W] -> Add5/1
  [DC_28V_Load] -> Enabled DC Load2/2
  DC Bus 1/3(IDC_2) -> Terminator3/1
  DC Bus 1/2(IDC_1) -> Terminator4/1
  DC Bus 3/2(IDC_1) -> Terminator5/1
  DC Bus 3/3(IDC_2) -> Terminator6/1
  Transformer-rectifier2/1 -> Terminator7/1
  Transformer-rectifier/1 -> Terminator8/1
  RPM/1 -> Generation Unit Sync-Sync4/1
  RPM1/1 -> Generation Unit Sync-Sync5/1
  Automatic Transformer Rectifier Unit/2(Iin) -> Scope14/1, Sum3/3
  Engine Outputs/1(Electrical) -> Terminator/1, Scope11/1
  Constant1/1 -> DC Bus 1/2(VDC_1)
  Product3/1 -> [AC230_Power]
  [AC230_Power] -> Add1/1
  Product/1 -> [DC270_Power]
  Product1/1 -> Scope16/1, [AC115_Power]
  Product2/1 -> [DC28_Power]
  [AC115_Power] -> Add1/2
  [DC270_Power] -> Add/1
  [DC28_Power] -> Add/2
  Automatic Transformer Rectifier Unit/1(Vout dqo) -> Product1/1, Scope8/1
  Constant/1 -> DC Bus 3/2(VDC_1)
  Constant5/1 -> Manual Switch/1
  Constant6/1 -> Manual Switch/2
  Memory3/1 -> 230 Vac Distr/7(I_Bus)
  Constant13/1 -> Enabled_AC_Loadloss1/2

== system Electrical787_Isolated_2013a/230 Vac Distr ==
  note: Generator Bus 1
  note: Generator Bus 2
  Gen 1 : Inport
  Gen 2 : Inport  Port=2
  Gen 3 : Inport  Port=3
  Gen 4 : Inport  Port=4
  Gen 5 : Inport  Port=5
  Gen 6 : Inport  Port=6
  I_Bus : Inport  Port=7
  Gain : Gain  Gain=1/2
  Gen Bus w/ APU switch : PowerFlowLib/Energy & Power Systems/Electrical/Systems/Gen Bus w// APU switch  LOWVLIMIT=90  UPVLIMIT=250  bus_st=2
  Gen Bus w/ APU switch1 : PowerFlowLib/Energy & Power Systems/Electrical/Systems/Gen Bus w// APU switch  LOWVLIMIT=90  UPVLIMIT=250  bus_st=2
  Terminator : Terminator
  Terminator1 : Terminator
  Vbus1 : Outport
  Vbus2 : Outport  Port=2
  tag scope: i_APU1=global, i_APU2=global, i_GND1=global, i_GND2=global, i_MAIN1=global, i_MAIN2=global
  wires:
  Gen Bus w/ APU switch/3 -> [i_APU1]
  Gen Bus w/ APU switch/4 -> [i_GND1]
  [Gen_Bus1] -> Gen Bus w/ APU switch/1
  Gen Bus w/ APU switch/2 -> [i_MAIN1]
  Gen Bus w/ APU switch1/3 -> [i_APU2]
  Gen Bus w/ APU switch1/4 -> [i_GND2]
  Gen Bus w/ APU switch1/2 -> [i_MAIN2]
  [Gen_Bus2] -> Gen Bus w/ APU switch1/1
  Gen 1/1 -> Gen Bus w/ APU switch/2
  Gen 3/1 -> Gen Bus w/ APU switch1/2
  Gen 5/1 -> Gen Bus w/ APU switch/3
  Gen 6/1 -> Gen Bus w/ APU switch1/3
  Gen Bus w/ APU switch/1 -> Vbus1/1
  Gen Bus w/ APU switch1/1 -> Vbus2/1
  I_Bus/1 -> Gain/1
  Gain/1 -> Gen Bus w/ APU switch1/6, Gen Bus w/ APU switch/6
  Gen 2/1 -> Terminator/1
  Gen 4/1 -> Terminator1/1

== system Electrical787_Isolated_2013a/Automatic Transformer Rectifier Unit ==
  Vin dqo : Inport
  Iout dqo : Inport  Port=2
  Constant : Constant  Value=[0.5 0.5 0.5]
  Demux : Demux  Outputs=3
  Demux1 : Demux  Outputs=3
  Gain : Gain  Gain=.5
  Mux1 : Mux  Inputs=3
  Mux2 : Mux  Inputs=3
  Three Phase Full Bridge Practical : PowerFlowLib/Energy & Power Systems/Electrical/Rectifiers/Three Phase Full Bridge Practical  C=100e-6  Rc=1
  abc to qd0 : PowerFlowLib/Energy & Power Systems/Electrical/Coordinate Transformation/abc to qd0
  qd0 to abc : PowerFlowLib/Energy & Power Systems/Electrical/Coordinate Transformation/qd0 to abc
  three-phase full-bridge inverter1 : PowerFlowLib/Energy & Power Systems/Electrical/Inverters/three-phase  full-bridge  inverter1
  Vout dqo : Outport
  Iin : Outport  Port=2
  wires:
  Three Phase Full Bridge Practical/1 -> three-phase full-bridge inverter1/2
  Constant/1 -> three-phase full-bridge inverter1/1
  three-phase full-bridge inverter1/1 -> Demux/1
  Demux/1 -> abc to qd0/1
  Demux/2 -> abc to qd0/2
  Demux/3 -> abc to qd0/3
  abc to qd0/1 -> Mux1/1
  abc to qd0/2 -> Mux1/2
  abc to qd0/3 -> Mux1/3
  three-phase full-bridge inverter1/2 -> Three Phase Full Bridge Practical/2
  Demux1/1 -> qd0 to abc/1
  Demux1/2 -> qd0 to abc/2
  Demux1/3 -> qd0 to abc/3
  qd0 to abc/1 -> Mux2/1
  qd0 to abc/2 -> Mux2/2
  qd0 to abc/3 -> Mux2/3
  Mux2/1 -> three-phase full-bridge inverter1/3
  Three Phase Full Bridge Practical/2 -> Iin/1
  Iout dqo/1 -> Demux1/1
  Vin dqo/1 -> Three Phase Full Bridge Practical/1
  Mux1/1 -> Gain/1
  Gain/1 -> Vout dqo/1

== system Electrical787_Isolated_2013a/Bus Controls ==
  Constant{1..5} (5 alike) : Constant
  Gen_Bus1 : Outport
  Gen_Bus2 : Outport  Port=2
  270V_DC_Bus : Outport  Port=3
  115V_AC_Bus : Outport  Port=4
  28V_DC_Bus : Outport  Port=5
  wires:
  Constant3/1 -> 28V_DC_Bus/1
  Constant5/1 -> 115V_AC_Bus/1
  Constant2/1 -> 270V_DC_Bus/1
  Constant4/1 -> Gen_Bus2/1
  Constant1/1 -> Gen_Bus1/1

== system Electrical787_Isolated_2013a/DC Bus 1 ==
  Select : Inport
  VDC_1 : Inport  Port=2
  VDC_2 : Inport  Port=3
  Load current : Inport  Port=4
  Compare To Constant : simulink/Logic and Bit Operations/Compare To Constant  relop=<=  const=3.0  OutDataTypeStr=boolean
  Compare To Constant1 : simulink/Logic and Bit Operations/Compare To Constant  relop=<=  const=3.0  OutDataTypeStr=boolean
  Constant : Constant  Value=[0]
  Multiport Switch : MultiPortSwitch  Inputs=2
  Switch : Switch  Criteria=u2 ~= 0
  Switch1 : Switch  Criteria=u2 ~= 0
  Vbus : Outport
  IDC_1 : Outport  Port=2
  IDC_2 : Outport  Port=3
  wires:
  Load current/1 -> Switch1/1, Switch/1
  Multiport Switch/1 -> Vbus/1
  VDC_1/1 -> Multiport Switch/2
  VDC_2/1 -> Multiport Switch/3
  Select/1 -> Multiport Switch/1, Compare To Constant/1, Compare To Constant1/1
  Compare To Constant/1 -> Switch/2
  Compare To Constant1/1 -> Switch1/2
  Constant/1 -> Switch/3, Switch1/3
  Switch/1 -> IDC_1/1
  Switch1/1 -> IDC_2/1

== system Electrical787_Isolated_2013a/DC Bus 3 ==
  Select : Inport
  VDC_1 : Inport  Port=2
  VDC_2 : Inport  Port=3
  Load current : Inport  Port=4
  Compare To Constant : simulink/Logic and Bit Operations/Compare To Constant  relop=<=  const=3.0  OutDataTypeStr=boolean
  Compare To Constant1 : simulink/Logic and Bit Operations/Compare To Constant  relop=<=  const=3.0  OutDataTypeStr=boolean
  Constant : Constant  Value=[0]
  Multiport Switch : MultiPortSwitch  Inputs=2
  Switch : Switch  Criteria=u2 ~= 0
  Switch1 : Switch  Criteria=u2 ~= 0
  Vbus : Outport
  IDC_1 : Outport  Port=2
  IDC_2 : Outport  Port=3
  wires:
  Load current/1 -> Switch1/1, Switch/1
  Multiport Switch/1 -> Vbus/1
  VDC_1/1 -> Multiport Switch/2
  VDC_2/1 -> Multiport Switch/3
  Select/1 -> Multiport Switch/1, Compare To Constant/1, Compare To Constant1/1
  Compare To Constant/1 -> Switch/2
  Compare To Constant1/1 -> Switch1/2
  Constant/1 -> Switch/3, Switch1/3
  Switch/1 -> IDC_1/1
  Switch1/1 -> IDC_2/1

== system Electrical787_Isolated_2013a/Enabled_AC_Loadloss ==
  Load Master Vector : Inport
  Vdq0 : Inport  Port=2
  Enable : EnablePort
  Enabled Subsystem : Subsystem  TreatAsAtomicUnit=on
  Enabled Subsystem1 : Subsystem  TreatAsAtomicUnit=on
  Scope : Scope
      settings: YMin=-18.75  YMax=168.75
  Scope1 : Scope
      settings: YMin=-10.27912  YMax=92.51202  SaveName=ScopeData2
  Sum1 : Sum  Inputs=|++
  Idq0 : Outport
  loss : Outport  Port=2
  wires:
  Enabled Subsystem/2(loss) -> loss/1
  Load Master Vector/1 -> Scope/1, Enabled Subsystem1/2(Ext vector)
  Sum1/1 -> Idq0/1
  Enabled Subsystem/1(Idq0) -> Sum1/2
  Enabled Subsystem1/1(Idq0) -> Sum1/1
  Vdq0/1 -> Enabled Subsystem1/1("Vdq0 "), Scope1/1, Enabled Subsystem/1("Vdq0 ")

== system Electrical787_Isolated_2013a/Engine Outputs ==
  Left_Wing_Toqrue_Nm : Inport
  Rght_Wing_Torque_Nm : Inport  Port=2
  APU_Torque_Nm : Inport  Port=3
  Bus Creator : BusCreator  Inputs=3
  Electrical : Outport
  wires:
  Rght_Wing_Torque_Nm/1 -> Bus Creator/2  "Right Wing Torq (Nm)"
  APU_Torque_Nm/1 -> Bus Creator/3  "APU Torq (Nm)"
  Left_Wing_Toqrue_Nm/1 -> Bus Creator/1  "Left Wing Torq (Nm)"
  Bus Creator/1 -> Electrical/1

== system Electrical787_Isolated_2013a/Generation Unit Sync-Sync1 ==
  engine speed : Inport
  idq0 : Inport  Port=2
  Temperature : Inport  Port=3
  Bus Creator : BusCreator  Inputs=3
  Bus Creator1 : BusCreator  Inputs=3
  Coeff of Resistance : Gain  Gain=3.85e-3
  Demux : Demux  Outputs=3
  Gain : Gain  Gain=200*2/3
  Gain1 : Gain  Gain=200
  Generator : Subsystem
      mask Display:
      | p = 0:0.1:(2*pi+0.1);
      | plot(sin(p), cos(p));
      | p1 = (-pi/8-0.1-0.2):0.1:(pi/8+0.1-0.2);
      | plot(0.8*sin(p1), 0.8*cos(p1), 0.8*sin(p1+pi), 0.8*cos(p1+pi));
      | p2 = sin((-pi/8-0.1-0.2+pi/8+0.1-0.2)/2);
      | p3 = sin((-pi/8-0.1-0.2+pi/8+0.1-0.2)/2+pi);
      | p4 = cos((-pi/8-0.1-0.2+pi/8+0.1-0.2)/2);
      | p5 = cos((-pi/8-0.1-0.2+pi/8+0.1-0.2)/2+pi);
      | plot(0.8*[p2, p3], 0.8*[p4, p5]);
      | port_label('output', 1, 'Vdq0');
      | port_label('output', 2, 'Te');
      | port_label('output', 3, 'Vfd');
      | port_label('output', 4, 'Ploss');
      | port_label('input', 1, 'idq0');
      | port_label('input', 2, 'w');
      | port_label('input', 3, 'ifd');
  Initial Temperature : Constant  Value=25
  Memory : Memory
  Permanent Magnet Synchronous Generator1 : PowerFlowLib/Energy & Power Systems/Electrical/Machines/Permanent Magnet Synchronous Generator1
  RPM_to_radps : Gain  Gain=pi/30
  Scope2 : Scope
      settings: TimeRange=100  YMin=0  YMax=5500
  Sum : Sum  Inputs=++|
  Sum1 : Sum
  Sum5 : Sum  Inputs=|+-
  Sum6 : Sum  Inputs=|++
  control1 : Constant
  data_sink : PowerFlowLib/Support Functions//Tools/data_sink
  one : Constant
  three-phase active rectifier Voltage Mode : PowerFlowLib/Energy & Power Systems/Electrical/Rectifiers/three-phase  active rectifier Voltage Mode  L=1  C=1e-4
  vdq0 : Outport
  engine torque : Outport  Port=2
  Ploss : Outport  Port=3
  wires:
  Temperature/1 -> Sum5/1
  Initial Temperature/1 -> Sum5/2
  Sum5/1 -> Coeff of Resistance/1
  Coeff of Resistance/1 -> Sum6/1
  one/1 -> Sum6/2
  Sum6/1 -> [R_temp_delta]
  Memory/1 -> Permanent Magnet Synchronous Generator1/1
  Sum1/1 -> Ploss/1, Bus Creator/2  "Ploss (W)"
  Generator/4(Ploss) -> Sum1/2
  Permanent Magnet Synchronous Generator1/3 -> Sum1/1
  Generator/1(vdq0) -> vdq0/1, Demux/1  "Vdq0 (V)"
  idq0/1 -> Generator/1(idq0)
  Generator/2(Te) -> Sum/2
  Permanent Magnet Synchronous Generator1/2 -> Sum/1
  three-phase active rectifier Voltage Mode/2 -> Memory/1
  three-phase active rectifier Voltage Mode/1 -> Gain/1
  Gain/1 -> Bus Creator/3, Generator/3(ifd')  "Excit current (A)"
  Gain1/1 -> three-phase active rectifier Voltage Mode/3
  Generator/3(vfd') -> Gain1/1
  control1/1 -> three-phase active rectifier Voltage Mode/2
  Permanent Magnet Synchronous Generator1/1 -> three-phase active rectifier Voltage Mode/1
  RPM_to_radps/1 -> Permanent Magnet Synchronous Generator1/2, Generator/2(w), Scope2/1
  Sum/1 -> engine torque/1
  Bus Creator/1 -> data_sink/1
  Demux/1 -> Bus Creator1/1  "vd"
  Demux/2 -> Bus Creator1/2  "vq"
  Demux/3 -> Bus Creator1/3  "v0"
  Bus Creator1/1 -> Bus Creator/1  "vdq0 (V)"
  engine speed/1 -> RPM_to_radps/1
  [R_temp_delta] -> Generator/4(Temp)
